simulink model "stg2_tv"  (Simulink 7.0)
settings: Solver=ode45  StartTime=0.0  StopTime=200000  RelTol=1e-3
undefined symbols (not defined in the file): pfb_coeff_gen_calc
libraries: xbsIndex_r4 x911, casper_library x87, xps_library x7
(part 1 of 12)
settings Model: Creator=dave  LastModifiedBy=dave

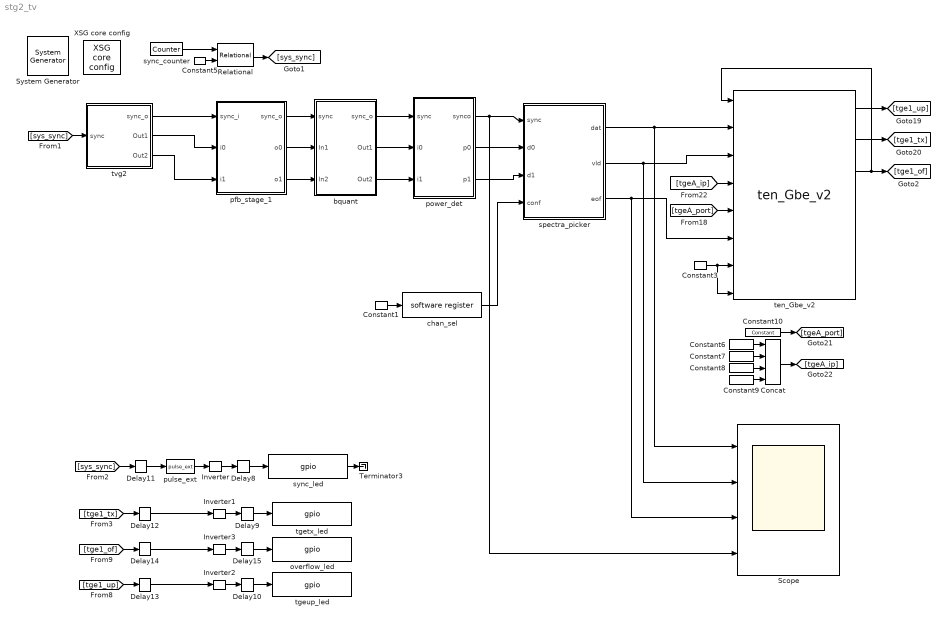
== system stg2_tv ==
  " System Generator" : xbsIndex_r4/ System Generator  Tag=genX  SystemSampleTime=-1  xilinxfamily=virtex5  part=xc5vlx110t  speed=-1  package=ff1136  synthesis_tool=XST  clock_wrapper=Clock Enables  directory=./qdr_cturn/sysgen  testbench=off  simulink_period=1  sysclk_period=8.3333  dcm_input_clock_period=100  incr_netlist=off  trim_vbits=Everywhere in SubSystem  dbl_ovrd=According to Block Masks  core_generation=According to Block Masks  run_coregen=off  deprecated_control=off  eval_field=0  block_type=sysgen
      settings: block_version=10.1.3
  Concat : xbsIndex_r4/Concat  num_inputs=4  dbl_ovrd=off  block_type=concat
      settings: block_version=10.1.3
  Constant1 : xbsIndex_r4/Constant  arith_type=Unsigned  const=4  n_bits=32  bin_pt=0  explicit_period=on  period=1  equ=P=C  opselect=C  inp2=PCIN>>17  opr=+  inp1=P  carry=CIN  dbl_ovrd=off  block_type=constant
  Constant10 : xbsIndex_r4/Constant  arith_type=Unsigned  const=10000  n_bits=16  bin_pt=0  explicit_period=off  period=1  equ=P=C  opselect=C  inp2=PCIN>>17  opr=+  inp1=P  carry=CIN  dbl_ovrd=off  block_type=constant
  Constant3 : xbsIndex_r4/Constant  arith_type=Boolean  const=0  n_bits=32  bin_pt=0  explicit_period=on  period=1  equ=P=C  opselect=C  inp2=PCIN>>17  opr=+  inp1=P  carry=CIN  dbl_ovrd=off  block_type=constant
  Constant5 : xbsIndex_r4/Constant  arith_type=Unsigned  const=0  n_bits=32  bin_pt=0  explicit_period=on  period=1  equ=P=C  opselect=C  inp2=PCIN>>17  opr=+  inp1=P  carry=CIN  dbl_ovrd=off  block_type=constant
  Constant6 : xbsIndex_r4/Constant  arith_type=Unsigned  const=192  n_bits=8  bin_pt=0  explicit_period=off  period=1  equ=P=C  opselect=C  inp2=PCIN>>17  opr=+  inp1=P  carry=CIN  dbl_ovrd=off  block_type=constant
  Constant7 : xbsIndex_r4/Constant  arith_type=Unsigned  const=168  n_bits=8  bin_pt=0  explicit_period=off  period=1  equ=P=C  opselect=C  inp2=PCIN>>17  opr=+  inp1=P  carry=CIN  dbl_ovrd=off  block_type=constant
  Constant8 : xbsIndex_r4/Constant  arith_type=Unsigned  const=5  n_bits=8  bin_pt=0  explicit_period=off  period=1  equ=P=C  opselect=C  inp2=PCIN>>17  opr=+  inp1=P  carry=CIN  dbl_ovrd=off  block_type=constant
  Constant9 : xbsIndex_r4/Constant  arith_type=Unsigned  const=2  n_bits=8  bin_pt=0  explicit_period=off  period=1  equ=P=C  opselect=C  inp2=PCIN>>17  opr=+  inp1=P  carry=CIN  dbl_ovrd=off  block_type=constant
  Delay{8..15} (8 alike) : xbsIndex_r4/Delay  en=off  latency=1  dbl_ovrd=off  reg_retiming=off  block_type=delay
  Inverter{,1..3} (4 alike) : xbsIndex_r4/Inverter  en=off  latency=0  dbl_ovrd=off  block_type=inv
  Relational : xbsIndex_r4/Relational  mode=a=b  en=off  latency=1  dbl_ovrd=off  block_type=relational
      settings: block_version=10.1.3
  Scope : Scope  NumInputPorts=4
      settings: YMin=-5~-5~-5~-5  YMax=5~5~5~5
  Terminator3 : Terminator
  XSG core config : xps_library/XSG core config  Tag=xps:xsg  SystemSampleTime=-1  hw_sys=ROACH:lx110t  ibob_linux=off  clk_src=sys_clk  iBOB_clk_src=sys_clk  BEE2_ctrl_clk_src=sys_clk  BEE2_usr_clk_src=sys_clk  ROACH_clk_src=sys_clk  CORR_clk_src=sys_clk  gpio_clk_io_group=iBOB:sma  gpio_clk_bit_index=0  clk_rate=100  sample_period=1  synthesis_tool=XST  mpc_type=powerpc440_ext
  bquant : Subsystem  mask{fact=8, bits=9}
      mask prompts: fact "fact (2^n)"; bits "quant bits"
  chan_sel : xps_library/software register  Tag=xps:sw_reg  SystemSampleTime=-1  io_dir=From Processor  arith_type=Unsigned  bitwidth=32  bin_pt=0  sample_period=1  gw_name=stg2_tv_chan_sel_user_data_out
      link override stg2_tv_chan_sel_user_data_out: arith_type=Unsigned  n_bits=32  bin_pt=0  period=1
  overflow_led : xps_library/gpio  Tag=xps:gpio  SystemSampleTime=-1  io_group=ROACH:led  io_dir=out  arith_type=Boolean  bitwidth=1  bin_pt=0  bit_index=2  sample_period=1  use_single_ended=off  use_ddr=off  reg_iob=on  reg_clk_phase=0  termination=None
      link override convert: arith_type=Boolean  n_bits=1  bin_pt=0
  pfb_stage_1 : Subsystem
  power_det : Subsystem
  pulse_ext : casper_library/Misc/pulse_ext  SystemSampleTime=-1  pulse_len=2^25
  spectra_picker : Subsystem
  sync_counter : xbsIndex_r4/Counter  cnt_type=Free Running  cnt_to=Inf  operation=Up  start_count=0  cnt_by_val=1  arith_type=Unsigned  n_bits=33  bin_pt=0  load_pin=off  rst=off  en=off  explicit_period=on  period=1  dbl_ovrd=off  use_behavioral_HDL=off  use_rpm=off  implementation=Fabric  block_type=counter
  sync_led : xps_library/gpio  Tag=xps:gpio  SystemSampleTime=-1  io_group=ROACH:led  io_dir=out  arith_type=Boolean  bitwidth=1  bin_pt=0  bit_index=0  sample_period=1  use_single_ended=off  use_ddr=off  reg_iob=on  reg_clk_phase=0  termination=None
      link override convert: arith_type=Boolean  n_bits=1  bin_pt=0
  ten_Gbe_v2 : xps_library/ten_Gbe_v2  Tag=xps:tengbe_v2  SystemSampleTime=-1  port=0  rx_dist_ram=on  show_param=on  pre_emph=3  swing=800  fab_en=on  fab_mac=hex2dec('123456780000')  fab_ip=192*(2^24) + 168*(2^16) + 5*(2^8) + 20*(2^0)  fab_udp=10000  fab_gate=1  cpu_rx_en=on  cpu_tx_en=on
  tgetx_led : xps_library/gpio  Tag=xps:gpio  SystemSampleTime=-1  io_group=ROACH:led  io_dir=out  arith_type=Boolean  bitwidth=1  bin_pt=0  bit_index=1  sample_period=1  use_single_ended=off  use_ddr=off  reg_iob=on  reg_clk_phase=0  termination=None
      link override convert: arith_type=Boolean  n_bits=1  bin_pt=0
  tgeup_led : xps_library/gpio  Tag=xps:gpio  SystemSampleTime=-1  io_group=ROACH:led  io_dir=out  arith_type=Boolean  bitwidth=1  bin_pt=0  bit_index=3  sample_period=1  use_single_ended=off  use_ddr=off  reg_iob=on  reg_clk_phase=0  termination=None
      link override convert: arith_type=Boolean  n_bits=1  bin_pt=0
  tvg2 : Subsystem
  wires:
  pulse_ext/1 -> Inverter/1
  [sys_sync] -> Delay11/1
  Delay8/1 -> sync_led/1
  Delay11/1 -> pulse_ext/1
  Inverter/1 -> Delay8/1
  sync_counter/1 -> Relational/1
  Constant5/1 -> Relational/2
  Relational/1 -> [sys_sync]
  sync_led/1 -> Terminator3/1
  [sys_sync] -> tvg2/1(sync)
  tvg2/1(sync_o) -> pfb_stage_1/1(sync_i)
  tvg2/2(Out1) -> pfb_stage_1/2(i0)
  tvg2/3(Out2) -> pfb_stage_1/3(i1)
  pfb_stage_1/1(sync_o) -> bquant/1(sync)
  pfb_stage_1/2(o0) -> bquant/2(In1)
  pfb_stage_1/3(o1) -> bquant/3(In2)
  bquant/1(sync_o) -> power_det/1(sync)
  bquant/2(Out1) -> power_det/2(i0)
  bquant/3(Out2) -> power_det/3(i1)
  Constant1/1 -> chan_sel/1
  ten_Gbe_v2/5 -> ten_Gbe_v2/1, [tge1_of]
  Constant6/1 -> Concat/1
  Constant7/1 -> Concat/2
  Constant8/1 -> Concat/3
  Constant9/1 -> Concat/4
  Concat/1 -> [tgeA_ip]
  Constant10/1 -> [tgeA_port]
  [tge1_tx] -> Delay12/1
  [tge1_up] -> Delay13/1
  Delay9/1 -> tgetx_led/1
  Delay10/1 -> tgeup_led/1
  Delay12/1 -> Inverter1/1
  Delay13/1 -> Inverter2/1
  Inverter1/1 -> Delay9/1
  Inverter2/1 -> Delay10/1
  Delay15/1 -> overflow_led/1
  Inverter3/1 -> Delay15/1
  [tge1_of] -> Delay14/1
  Delay14/1 -> Inverter3/1
  [tgeA_ip] -> ten_Gbe_v2/4
  [tgeA_port] -> ten_Gbe_v2/5
  Constant3/1 -> ten_Gbe_v2/7, ten_Gbe_v2/8
  ten_Gbe_v2/1 -> [tge1_up]
  ten_Gbe_v2/3 -> [tge1_tx]
  power_det/1(synco) -> spectra_picker/1(sync), Scope/4
  power_det/2(p0) -> spectra_picker/2(d0)
  power_det/3(p1) -> spectra_picker/3(d1)
  chan_sel/1 -> spectra_picker/4(conf)
  spectra_picker/1(dat) -> ten_Gbe_v2/2, Scope/1
  spectra_picker/2(vld) -> ten_Gbe_v2/3, Scope/2
  spectra_picker/3(eof) -> ten_Gbe_v2/6, Scope/3

== system stg2_tv/bquant ==
  sync : Inport
  In1 : Inport  Port=2
  In2 : Inport  Port=3
  Convert{,1..3} (4 alike) : xbsIndex_r4/Convert  arith_type="Signed  (2's comp)"  n_bits=bits  bin_pt=bits-1  quantization="Round  (unbiased: +/- Inf)"  overflow=Saturate  latency=0  dbl_ovrd=off  pipeline=off  block_type=convert
      settings: block_version=10.1.3
  Delay{1..5,7} (6 alike) : xbsIndex_r4/Delay  en=off  latency=1  dbl_ovrd=off  reg_retiming=off  block_type=delay
  Shift{,1..3} (4 alike) : xbsIndex_r4/Shift  shift_dir=Left  shift_bits=fact  en=off  latency=1  precision=Full  arith_type="Signed  (2's comp)"  n_bits=16  bin_pt=14  quantization=Truncate  overflow=Wrap  dbl_ovrd=off  block_type=shift
      settings: block_version=10.1.3
  c_to_ri : casper_library/Misc/c_to_ri  SystemSampleTime=-1  n_bits=25  bin_pt=24
      settings: AttributesFormatString=25_24 r/i
  c_to_ri1 : casper_library/Misc/c_to_ri  SystemSampleTime=-1  n_bits=25  bin_pt=24
      settings: AttributesFormatString=25_24 r/i
  ri_to_c : casper_library/Misc/ri_to_c  SystemSampleTime=-1
  ri_to_c1 : casper_library/Misc/ri_to_c  SystemSampleTime=-1
  sync_o : Outport
  Out1 : Outport  Port=2
  Out2 : Outport  Port=3
  wires:
  Delay3/1 -> sync_o/1
  Delay5/1 -> Delay3/1
  sync/1 -> Delay5/1
  ri_to_c1/1 -> Out2/1
  In2/1 -> c_to_ri1/1
  ri_to_c/1 -> Out1/1
  In1/1 -> c_to_ri/1
  Delay7/1 -> ri_to_c1/2
  Delay4/1 -> ri_to_c1/1
  Delay2/1 -> ri_to_c/2
  Delay1/1 -> ri_to_c/1
  Convert3/1 -> Delay7/1
  Convert2/1 -> Delay4/1
  Convert1/1 -> Delay2/1
  Convert/1 -> Delay1/1
  c_to_ri1/2 -> Shift3/1
  c_to_ri1/1 -> Shift2/1
  Shift3/1 -> Convert3/1
  Shift2/1 -> Convert2/1
  c_to_ri/2 -> Shift1/1
  c_to_ri/1 -> Shift/1
  Shift1/1 -> Convert1/1
  Shift/1 -> Convert/1

== system stg2_tv/pfb_stage_1 ==
  sync_i : Inport
  i0 : Inport  Port=2
  i1 : Inport  Port=3
  " window" : Subsystem  mask{wintype=0, size=10, coeff_width=18, o_width=25, i_width=9}
      mask prompts: wintype "Windowing Function:"; size "size (2^n)"; coeff_width "coeff width"; o_width "out width"; i_width "in width"
  Constant4 : xbsIndex_r4/Constant  arith_type=Unsigned  const=1023  n_bits=10  bin_pt=0  explicit_period=on  period=1  equ=P=C  opselect=C  inp2=PCIN>>17  opr=+  inp1=P  carry=CIN  dbl_ovrd=off  block_type=constant
  Delay{,1..3} (4 alike) : xbsIndex_r4/Delay  en=off  latency=1  dbl_ovrd=off  reg_retiming=off  block_type=delay
  Shift{1..4} (4 alike) : xbsIndex_r4/Shift  shift_dir=Right  shift_bits=1  en=off  latency=1  precision=Full  arith_type="Signed  (2's comp)"  n_bits=16  bin_pt=14  quantization=Truncate  overflow=Wrap  dbl_ovrd=off  block_type=shift
      settings: block_version=10.1.3
  c_to_ri : casper_library/Misc/c_to_ri  SystemSampleTime=-1  n_bits=25  bin_pt=24
      settings: AttributesFormatString=25_24 r/i
  c_to_ri1 : casper_library/Misc/c_to_ri  SystemSampleTime=-1  n_bits=25  bin_pt=24
      settings: AttributesFormatString=25_24 r/i
  fft : Subsystem  AncestorBlock=casper_library/FFTs/fft  mask(fft){FFTSize=10, input_bit_width=25, coeff_bit_width=18, n_inputs=0, quantization=Truncate, overflow=Wrap, add_latency=1, mult_latency=3, bram_latency=3, arch=Virtex5, opt_target=Multipliers, coeffs_bit_limit=8, delays_bit_limit=9, specify_mult=off, mult_spec=[0 1 1 2 1 1 1 1 1 1]}
      mask prompts: FFTSize "Size of FFT: (2^?)"; input_bit_width "Input/Output Bit Width"; coeff_bit_width "Coefficient Bit Width"; n_inputs "Number of Simultaneous Inputs: (2^?)"; quantization "Quantization Behavior"; overflow "Overflow Behavior"; add_latency "Add Latency"; mult_latency "Mult Latency"; bram_latency "BRAM Latency"; arch "Architecture"; opt_target "Optimisation Target"; coeffs_bit_limit "Number bits above which to store stage's coefficients in BRAM (2^? bits)"; delays_bit_limit "Number bits above which to store stage's delays in BRAM (2^? bits)"; specify_mult "Specify multiplier use (behavioral HDL if not specified)"; mult_spec "Multiplier specification (0=core, 1=embedded, 2=behavioural) (left=1st stage)"
      mask init:
      | fft_init(gcb,...
      |     'FFTSize', FFTSize, ...
      |     'input_bit_width', input_bit_width, ...
      |     'coeff_bit_width', coeff_bit_width, ...
      |     'n_inputs', n_inputs, ...
      |     'quantization', quantization, ...
      |     'overflow', overflow, ...
      |     'add_latency', add_latency, ...
      |     'mult_latency', mult_latency, ...
      |     'bram_latency', bram_latency, ...
      |     'arch', arch, ...
      |     'opt_target', opt_target, ...
      |     'coeffs_bit_limit', coeffs_bit_limit, ...
      |     'delays_bit_limit', delays_bit_limit, ...
      |     'specify_mult', specify_mult, ...
      |     'mult_spec', mult_spec);
      settings: AttributesFormatString=FFTSize=10, n_inputs=0
      mask Help: eval('xlWeb([getenv(''MLIB_ROOT''), ''\doc\htmlblocks\sp_fft\sp_fft.html''])')
      mask StyleString: edit,edit,edit,edit,popup(Truncate|Round  (unbiased: +/- Inf)|Round  (unbiased: Even Values)),popup(Wrap|Saturate|Error),edit,edit,edit,popup(Virtex2Pro|Virtex5),popup(Logic|Multipliers),edit,edit,checkbox,edit
      mask CallbackString:
      | % fft_size = eval(get_param(gcb, 'FFTSize'));
      | % old_vec = eval(get_param(gcb, 'mult_spec'));
      | 
      | % vec = 2.*ones(1,fft_size);
      | % old_size = length(old_vec);
      | 
      | % if(old_size <= fft_size), size = old_size;
      | % else, size = fft_size;
      | % end
      | 
      | % for n = 1:size, vec(n) = old_vec(n); end
      | % set_param(gcb, 'mult_spec', mat2str(vec));|||||||||||||specify_mult = get_param(gcb,'specify_mult');
      | visibs = get_param(gcb, 'MaskVisibilities');
      | if( strcmp(specify_mult,'off')), visibs{15} = 'off';
      | else visibs{15} = 'on';
      | end
      | set_param(gcb, 'MaskVisibilities', visibs);
      | 
      | |% vec = eval( get_param(gcb, 'mult_spec'));
      | % vec_size = length(vec);
      | % fft_size = eval( get_param(gcb, 'FFTSize'));
      | % new_vec = 2.*ones(1, fft_size);
      | 
      | % if(vec_size <= fft_size), size = vec_size;
      | % else size = fft_size;
      | % end
      | 
      | % for n=1:size,
      | %    new_vec(n) = vec(n);
      | % end
      | % set_param(gcb, 'mult_spec', mat2str(new_vec));
  ri_to_c : casper_library/Misc/ri_to_c  SystemSampleTime=-1
  ri_to_c1 : casper_library/Misc/ri_to_c  SystemSampleTime=-1
  sync_o : Outport
  o0 : Outport  Port=2
  o1 : Outport  Port=3
  wires:
  " window"/3(pol1_o) -> c_to_ri1/1
  " window"/2(pol0_o) -> c_to_ri/1
  " window"/1(sync_o) -> Delay/1
  ri_to_c1/1 -> Delay3/1
  Shift2/1 -> ri_to_c1/2
  Shift4/1 -> ri_to_c1/1
  c_to_ri1/2 -> Shift2/1
  c_to_ri1/1 -> Shift4/1
  ri_to_c/1 -> Delay2/1
  Shift1/1 -> ri_to_c/2
  Shift3/1 -> ri_to_c/1
  c_to_ri/2 -> Shift1/1
  c_to_ri/1 -> Shift3/1
  Delay/1 -> Delay1/1
  sync_i/1 -> " window"/1(sync)
  fft/3(out1) -> o1/1
  fft/2(out0) -> o0/1
  fft/1(sync_out) -> sync_o/1
  Constant4/1 -> fft/2(shift)
  i1/1 -> " window"/3(pol1_i)
  i0/1 -> " window"/2(pol0_i)
  Delay1/1 -> fft/1(sync)
  Delay2/1 -> fft/3(pol0)
  Delay3/1 -> fft/4(pol1)

== system stg2_tv/power_det ==
  sync : Inport
  i0 : Inport  Port=2
  i1 : Inport  Port=3
  Delay2 : xbsIndex_r4/Delay  en=off  latency=3  dbl_ovrd=off  reg_retiming=off  block_type=delay
  power0 : casper_library/Misc/power  SystemSampleTime=-1  BitWidth=9  add_latency=1  mult_latency=2
  power1 : casper_library/Misc/power  SystemSampleTime=-1  BitWidth=9  add_latency=1  mult_latency=2
  synco : Outport
  p0 : Outport  Port=2
  p1 : Outport  Port=3
  wires:
  Delay2/1 -> synco/1
  sync/1 -> Delay2/1
  power1/1 -> p1/1
  i1/1 -> power1/1
  power0/1 -> p0/1
  i0/1 -> power0/1

== system stg2_tv/spectra_picker ==
  sync : Inport
  d0 : Inport  Port=2
  d1 : Inport  Port=3
  conf : Inport  Port=4
  Constant2 : xbsIndex_r4/Constant  arith_type=Unsigned  const=2^10-1  n_bits=10  bin_pt=0  explicit_period=on  period=1  equ=P=C  opselect=C  inp2=PCIN>>17  opr=+  inp1=P  carry=CIN  dbl_ovrd=off  block_type=constant
  Delay{,1..4} (5 alike) : xbsIndex_r4/Delay  en=off  latency=1  dbl_ovrd=off  reg_retiming=off  block_type=delay
  Logical : xbsIndex_r4/Logical  logical_function=AND  inputs=2  en=off  latency=0  precision=Full  arith_type=Unsigned  n_bits=16  bin_pt=0  align_bp=on  dbl_ovrd=off  block_type=logical
  Mux : xbsIndex_r4/Mux  inputs=2  en=off  latency=0  precision=Full  arith_type=Unsigned  n_bits=16  bin_pt=14  quantization=Truncate  overflow=Wrap  dbl_ovrd=off  block_type=mux
  Relational1 : xbsIndex_r4/Relational  mode=a=b  en=off  latency=1  dbl_ovrd=off  block_type=relational
      settings: block_version=10.1.3
  Relational2 : xbsIndex_r4/Relational  mode=a=b  en=off  latency=1  dbl_ovrd=off  block_type=relational
      settings: block_version=10.1.3
  Slice : xbsIndex_r4/Slice  nbits=9  boolean_output=off  mode=Lower Bit Location + Width  bit1=0  base1=LSB of Input  bit0=1  base0=LSB of Input  dbl_ovrd=off  block_type=slice
      settings: infoedit="Extracts a given range of bits from each input sample and presents it at the output.  The output type is ordinarily unsigned with binary point at zero, but can be Boolean when the slice is one bit wide.<P><P>Hardware notes: In hardware this block costs nothing."  block_version=10.1.3
  Slice1 : xbsIndex_r4/Slice  nbits=1  boolean_output=off  mode=Lower Bit Location + Width  bit1=0  base1=LSB of Input  bit0=0  base0=LSB of Input  dbl_ovrd=off  block_type=slice
      settings: infoedit="Extracts a given range of bits from each input sample and presents it at the output.  The output type is ordinarily unsigned with binary point at zero, but can be Boolean when the slice is one bit wide.<P><P>Hardware notes: In hardware this block costs nothing."  block_version=10.1.3
  Slice2 : xbsIndex_r4/Slice  nbits=9  boolean_output=off  mode=Lower Bit Location + Width  bit1=0  base1=LSB of Input  bit0=10  base0=LSB of Input  dbl_ovrd=off  block_type=slice
      settings: infoedit="Extracts a given range of bits from each input sample and presents it at the output.  The output type is ordinarily unsigned with binary point at zero, but can be Boolean when the slice is one bit wide.<P><P>Hardware notes: In hardware this block costs nothing."  block_version=10.1.3
  Slice3 : xbsIndex_r4/Slice  nbits=10  boolean_output=off  mode=Lower Bit Location + Width  bit1=0  base1=LSB of Input  bit0=0  base0=LSB of Input  dbl_ovrd=off  block_type=slice
      settings: infoedit="Extracts a given range of bits from each input sample and presents it at the output.  The output type is ordinarily unsigned with binary point at zero, but can be Boolean when the slice is one bit wide.<P><P>Hardware notes: In hardware this block costs nothing."  block_version=10.1.3
  frame_counter : xbsIndex_r4/Counter  cnt_type=Free Running  cnt_to=Inf  operation=Up  start_count=0  cnt_by_val=1  arith_type=Unsigned  n_bits=19  bin_pt=0  load_pin=off  rst=on  en=off  explicit_period=on  period=1  dbl_ovrd=off  use_behavioral_HDL=off  use_rpm=off  implementation=Fabric  block_type=counter
  dat : Outport
  vld : Outport  Port=2
  eof : Outport  Port=3
  wires:
  Delay/1 -> Slice/1, Slice1/1
  Slice1/1 -> Mux/1
  frame_counter/1 -> Slice2/1, Slice3/1
  Slice2/1 -> Relational1/1
  Slice/1 -> Relational1/2
  Mux/1 -> Delay1/1
  Slice3/1 -> Relational2/1
  Constant2/1 -> Relational2/2
  Relational2/1 -> Logical/1
  Relational1/1 -> Logical/2, Delay3/1
  Logical/1 -> Delay2/1
  Delay1/1 -> Delay4/1
  sync/1 -> frame_counter/1
  d0/1 -> Mux/2
  d1/1 -> Mux/3
  Delay2/1 -> eof/1
  Delay3/1 -> vld/1
  conf/1 -> Delay/1
  Delay4/1 -> dat/1

== system stg2_tv/tvg2 ==
  sync : Inport  OutDataType=sfix(16)  OutScaling=2^0
  Constant : xbsIndex_r4/Constant  arith_type=Signed (2's comp)  const=0  n_bits=9  bin_pt=8  explicit_period=on  period=1  equ=P=C  opselect=C  inp2=PCIN>>17  opr=+  inp1=P  carry=CIN  dbl_ovrd=off  block_type=constant
  Delay : xbsIndex_r4/Delay  en=off  latency=1  dbl_ovrd=off  reg_retiming=off  block_type=delay
  Delay1 : xbsIndex_r4/Delay  en=off  latency=1  dbl_ovrd=off  reg_retiming=off  block_type=delay
  Delay2 : xbsIndex_r4/Delay  en=off  latency=3  dbl_ovrd=off  reg_retiming=off  block_type=delay
  Delay3 : xbsIndex_r4/Delay  en=off  latency=1  dbl_ovrd=off  reg_retiming=off  block_type=delay
  Delay4 : xbsIndex_r4/Delay  en=off  latency=2  dbl_ovrd=off  reg_retiming=off  block_type=delay
  Mult : xbsIndex_r4/Mult  precision=User Defined  arith_type=Unsigned  n_bits=12  bin_pt=0  quantization=Truncate  overflow=Wrap  en=off  latency=3  dbl_ovrd=off  use_behavioral_HDL=off  use_embedded=on  opt=Speed  optimum_pipeline=off  pipeline=on  use_rpm=on  placement_style=Triangular  block_type=mult
      settings: infoedit=Hardware notes: To use the internal pipeline stage of the dedicated multiplier you must select 'Pipeline for maximum performance'.  block_version=10.1.3
  Shift : xbsIndex_r4/Shift  shift_dir=Right  shift_bits=6  en=off  latency=1  precision=User Defined  arith_type="Signed  (2's comp)"  n_bits=9  bin_pt=8  quantization="Round  (unbiased: +/- Inf)"  overflow=Wrap  dbl_ovrd=off  block_type=shift
      settings: block_version=10.1.3
  chan_s : xbsIndex_r4/Slice  nbits=9  boolean_output=off  mode=Lower Bit Location + Width  bit1=0  base1=LSB of Input  bit0=10  base0=LSB of Input  dbl_ovrd=off  block_type=slice
      settings: infoedit="Extracts a given range of bits from each input sample and presents it at the output.  The output type is ordinarily unsigned with binary point at zero, but can be Boolean when the slice is one bit wide.<P><P>Hardware notes: In hardware this block costs nothing."  block_version=10.1.3
  chan_s1 : xbsIndex_r4/Slice  nbits=10  boolean_output=off  mode=Lower Bit Location + Width  bit1=0  base1=LSB of Input  bit0=0  base0=LSB of Input  dbl_ovrd=off  block_type=slice
      settings: infoedit="Extracts a given range of bits from each input sample and presents it at the output.  The output type is ordinarily unsigned with binary point at zero, but can be Boolean when the slice is one bit wide.<P><P>Hardware notes: In hardware this block costs nothing."  block_version=10.1.3
  progress : xbsIndex_r4/Counter  cnt_type=Free Running  cnt_to=Inf  operation=Up  start_count=0  cnt_by_val=1  arith_type=Unsigned  n_bits=19  bin_pt=0  load_pin=off  rst=on  en=off  explicit_period=on  period=1  dbl_ovrd=off  use_behavioral_HDL=off  use_rpm=off  implementation=Fabric  block_type=counter
  ri_to_c : casper_library/Misc/ri_to_c  SystemSampleTime=-1
  ri_to_c1 : casper_library/Misc/ri_to_c  SystemSampleTime=-1
  tvg_lookup : xbsIndex_r4/ROM  depth=4096  initVector=cos(pi*(0:4065)/128)  distributed_mem=Block RAM  rst=off  init_reg=0  en=off  latency=2  arith_type="Signed  (2's comp)"  n_bits=9  bin_pt=8  dbl_ovrd=off  optimize=Area  use_rpm=on  block_type=sprom
      settings: block_version=10.1.3
  sync_o : Outport
  Out1 : Outport  Port=2
  Out2 : Outport  Port=3
  wires:
  progress/1 -> chan_s/1, chan_s1/1
  chan_s/1 -> [chan]
  chan_s1/1 -> [samp]
  ri_to_c/1 -> Out1/1
  ri_to_c1/1 -> Out2/1
  Constant/1 -> ri_to_c/2, ri_to_c1/1
  tvg_lookup/1 -> Shift/1
  Delay/1 -> ri_to_c/1, ri_to_c1/2
  sync/1 -> progress/1, Delay2/1
  Delay3/1 -> Delay1/1
  Delay1/1 -> sync_o/1
  [chan] -> Mult/1
  [samp] -> Mult/2
  Mult/1 -> tvg_lookup/1
  Delay2/1 -> Delay4/1
  Shift/1 -> Delay/1
  Delay4/1 -> Delay3/1

== system stg2_tv/pfb_stage_1/ window ==
  sync : Inport
  pol0_i : Inport  Port=2
  pol1_i : Inport  Port=3
  Delay : xbsIndex_r4/Delay  en=off  latency=2  dbl_ovrd=off  reg_retiming=off  block_type=delay
  Delay1 : xbsIndex_r4/Delay  en=off  latency=3  dbl_ovrd=off  reg_retiming=off  block_type=delay
  Mult{,1..3} (4 alike) : xbsIndex_r4/Mult  precision=Full  arith_type="Signed  (2's comp)"  n_bits=16  bin_pt=14  quantization=Truncate  overflow=Wrap  en=off  latency=3  dbl_ovrd=off  use_behavioral_HDL=off  use_embedded=on  opt=Speed  optimum_pipeline=off  pipeline=on  use_rpm=on  placement_style=Triangular  block_type=mult
      settings: infoedit=Hardware notes: To use the internal pipeline stage of the dedicated multiplier you must select 'Pipeline for maximum performance'.  block_version=10.1.3
  c_to_ri : casper_library/Misc/c_to_ri  SystemSampleTime=-1  n_bits=i_width  bin_pt=i_width-1
      settings: AttributesFormatString=9_8 r/i
  c_to_ri1 : casper_library/Misc/c_to_ri  SystemSampleTime=-1  n_bits=i_width  bin_pt=i_width-1
      settings: AttributesFormatString=9_8 r/i
  lookup_cntr : xbsIndex_r4/Counter  cnt_type=Free Running  cnt_to=Inf  operation=Up  start_count=0  cnt_by_val=1  arith_type=Unsigned  n_bits=size  bin_pt=0  load_pin=off  rst=on  en=off  explicit_period=on  period=1  dbl_ovrd=off  use_behavioral_HDL=off  use_rpm=off  implementation=Fabric  block_type=counter
  ri_to_c : casper_library/Misc/ri_to_c  SystemSampleTime=-1
  ri_to_c1 : casper_library/Misc/ri_to_c  SystemSampleTime=-1
  window_lookup : xbsIndex_r4/ROM  depth=2^size  initVector=pfb_coeff_gen_calc(size, 1,'hamming',0, 0,1,1)  distributed_mem=Block RAM  rst=off  init_reg=0  en=off  latency=2  arith_type="Signed  (2's comp)"  n_bits=18  bin_pt=17  dbl_ovrd=off  optimize=Area  use_rpm=on  block_type=sprom
      settings: block_version=10.1.3
  sync_o : Outport
  pol0_o : Outport  Port=2
  pol1_o : Outport  Port=3
  wires:
  Delay/1 -> Delay1/1
  lookup_cntr/1 -> window_lookup/1
  sync/1 -> lookup_cntr/1, Delay/1
  pol0_i/1 -> c_to_ri/1
  window_lookup/1 -> Mult/1, Mult1/1, Mult2/1, Mult3/1
  c_to_ri/1 -> Mult/2
  c_to_ri/2 -> Mult1/2
  Delay1/1 -> sync_o/1
  Mult/1 -> ri_to_c/1
  Mult1/1 -> ri_to_c/2
  Mult2/1 -> ri_to_c1/1
  Mult3/1 -> ri_to_c1/2
  pol1_i/1 -> c_to_ri1/1
  c_to_ri1/1 -> Mult2/2
  c_to_ri1/2 -> Mult3/2
  ri_to_c/1 -> pol0_o/1
  ri_to_c1/1 -> pol1_o/1

== system stg2_tv/pfb_stage_1/fft ==
  sync : Inport  OutDataType=sfix(16)  OutScaling=2^0
  shift : Inport  Port=2  OutDataType=sfix(16)  OutScaling=2^0
  pol0 : Inport  Port=3
  pol1 : Inport  Port=4
  fft_biplex0 : Subsystem  AncestorBlock=casper_library/FFTs/fft_biplex  mask(fft_biplex){FFTSize=10, input_bit_width=25, coeff_bit_width=18, quantization=Truncate, overflow=Wrap, add_latency=1, mult_latency=3, bram_latency=3, arch=Virtex5, opt_target=Multipliers, coeffs_bit_limit=8, delays_bit_limit=9, specify_mult=off, mult_spec=[2 2 2 2 2 2 2 2 2 2]}
      mask prompts: FFTSize "Size of FFT: (2^? pnts)"; input_bit_width "Input/Output Bit Width"; coeff_bit_width "Coefficient Bit Width"; quantization "Quantization Behavior"; overflow "Overflow Behavior"; add_latency "Add Latency"; mult_latency "Mult Latency"; bram_latency "BRAM Latency"; arch "Architecture"; opt_target "Optimisation Target"; coeffs_bit_limit "Number bits above which to store stage's coefficients in BRAM (2^? bits)"; delays_bit_limit "Number bits above which to implent stage's delays in BRAM (2^? bits)"; specify_mult "Specify multiplier use (behavioral HDL if not specified)"; mult_spec "Multiplier specification (0=core, 1=embedded, 2=behavioural) (left=1st stage)"
      mask init:
      | fft_biplex_init(gcb,...
      |     'FFTSize', FFTSize,...
      |     'input_bit_width', input_bit_width,...
      |     'coeff_bit_width', coeff_bit_width,...
      |     'quantization', quantization,...
      |     'overflow', overflow,...
      |     'add_latency', add_latency,...
      |     'mult_latency', mult_latency,...
      |     'bram_latency', bram_latency,...
      |     'arch', arch, ...
      |     'opt_target', opt_target, ...
      |     'coeffs_bit_limit', coeffs_bit_limit, ...
      |     'delays_bit_limit', delays_bit_limit, ...
      |     'specify_mult', specify_mult,...
      |     'mult_spec', mult_spec);
      settings: AttributesFormatString=|
      | FFTSize=10,
      |  arch=Virtex5,
      |  opt_target=Multipliers
      mask StyleString: edit,edit,edit,popup(Truncate|Round  (unbiased: +/- Inf)|Round  (unbiased: Even Values)),popup(Wrap|Saturate|Error),edit,edit,edit,popup(Virtex2Pro|Virtex5),popup(Logic|Multipliers),edit,edit,checkbox,edit
      mask CallbackString:
      | % fft_size = eval(get_param(gcb, 'FFTSize'));
      | % old_vec = eval(get_param(gcb, 'mult_spec'));
      | 
      | % vec = 2.*ones(1,fft_size);
      | % old_size = length(old_vec);
      | 
      | % if(old_size <= fft_size),
      | %    size = old_size;
      | % else,
      | %     size = fft_size;
      | % end
      | 
      | % for n = 1:size, vec(n) = old_vec(n); end
      | % set_param(gcb, 'mult_spec', mat2str(vec));||||||||||||specify_mult = get_param(gcb,'specify_mult');
      | visibs = get_param(gcb, 'MaskVisibilities');
      | 
      | if( strcmp(specify_mult,'off')), visibs{14} = 'off';
      | else, visibs{14} = 'on';
      | end
      | set_param(gcb, 'MaskVisibilities', visibs);
      | |% vec = eval( get_param(gcb, 'mult_spec'));
      | % vec_size = length(vec);
      | % fft_size = eval( get_param(gcb, 'FFTSize'));
      | % new_vec = 2.*ones(1, fft_size);
      | 
      | % if(vec_size <= fft_size), size = vec_size;
      | % else size = fft_size;
      | % end
      | 
      | % for n=1:size
      | %     new_vec(n) = vec(n);
      | % end
      | % set_param(gcb, 'mult_spec', mat2str(new_vec));
  sync_out : Outport
  out0 : Outport  Port=2
  out1 : Outport  Port=3
  of : Outport  Port=4
  wires:
  pol0/1 -> fft_biplex0/1(pol1)
  pol1/1 -> fft_biplex0/2(pol2)
  shift/1 -> fft_biplex0/4(shift)
  sync/1 -> fft_biplex0/3(sync)
  fft_biplex0/1(pol1_out) -> out0/1
  fft_biplex0/2(pol2_out) -> out1/1
  fft_biplex0/4(sync_out) -> sync_out/1
  fft_biplex0/3(of) -> of/1

== system stg2_tv/pfb_stage_1/fft/fft_biplex0 ==
  pol1 : Inport  OutDataType=sfix(16)  OutScaling=2^0
  pol2 : Inport  Port=2  OutDataType=sfix(16)  OutScaling=2^0
  sync : Inport  Port=3  OutDataType=sfix(16)  OutScaling=2^0
  shift : Inport  Port=4  OutDataType=sfix(16)  OutScaling=2^0
  biplex_core : Subsystem  AncestorBlock=casper_library/FFTs/biplex_core  mask(biplex_core){FFTSize=10, input_bit_width=25, coeff_bit_width=18, quantization=Truncate, overflow=Wrap, add_latency=1, mult_latency=3, bram_latency=3, arch=Virtex5, opt_target=Multipliers, coeffs_bit_limit=8, delays_bit_limit=9, specify_mult=off, mult_spec=[2 2 2 2 2 2 2 2 2 2]}
      mask prompts: FFTSize "Size of FFT: (2^? pnts)"; input_bit_width "Input/Output Bit Width"; coeff_bit_width "Coefficient Bit Width"; quantization "Quantization Behavior"; overflow "Overflow Behavior"; add_latency "Add Latency"; mult_latency "Mult Latency"; bram_latency "BRAM Latency"; arch "Architecture"; opt_target "Optimisation Target"; coeffs_bit_limit "Number bits above which to store stage's coefficients in BRAM (2^? bits)"; delays_bit_limit "Number bits above which to implent stage's delays in BRAM (2^? bits)"; specify_mult "Specify multiplier use (behavioural HDL if not specified)"; mult_spec "Multiplier specification (0=core, 1=embedded, 2=behavioural) (left=1st stage)"
      mask init:
      | biplex_core_init(gcb,...
      |     'FFTSize', FFTSize,...
      |     'input_bit_width', input_bit_width,...
      |     'coeff_bit_width', coeff_bit_width,...
      |     'quantization', quantization,...
      |     'overflow', overflow,...
      |     'add_latency', add_latency,...
      |     'mult_latency', mult_latency,...
      |     'bram_latency', bram_latency,...
      |     'arch', arch, ...
      |     'opt_target', opt_target, ...
      |     'coeffs_bit_limit', coeffs_bit_limit, ...
      |     'delays_bit_limit', delays_bit_limit, ...
      |     'specify_mult', specify_mult,...
      |     'mult_spec', mult_spec);
      settings: AttributesFormatString=|
      | FFTSize=10,
      |  opt_target=Multipliers,
      |  arch=Virtex5
      mask StyleString: edit,edit,edit,popup(Truncate|Round  (unbiased: +/- Inf)|Round  (unbiased: Even Values)),popup(Wrap|Saturate|Error),edit,edit,edit,popup(Virtex2Pro|Virtex5),popup(Logic|Multipliers),edit,edit,checkbox,edit
      mask CallbackString:
      | fft_size = eval(get_param(gcb, 'FFTSize'));
      | old_vec = eval(get_param(gcb, 'mult_spec'));
      | 
      | vec = 2.*ones(1,fft_size);
      | old_size = length(old_vec);
      | 
      | if(old_size <= fft_size),
      |     size = old_size;
      | else,
      |     size = fft_size;
      | end
      | 
      | for n = 1:size, vec(n) = old_vec(n); end
      | set_param(gcb, 'mult_spec', mat2str(vec));||||||||||||specify_mult = get_param(gcb,'specify_mult');
      | visibs = get_param(gcb,'MaskVisibilities');
      | if( strcmp(specify_mult,'off')), visibs{14} = 'off';
      | else, visibs{14} = 'on';
      | end
      | set_param(gcb, 'MaskVisibilities', visibs);
      | enables = get_param(gcb,'MaskVisibilities');
      | enables{14} = 'on';
      | set_param(gcb, 'MaskEnables', enables);
      | |vec = eval( get_param(gcb, 'mult_spec'));
      | vec_size = length(vec);
      | fft_size = eval( get_param(gcb, 'FFTSize'));
      | new_vec = 2.*ones(1, fft_size);
      | 
      | if(vec_size <= fft_size), size = vec_size;
      | else size = fft_size;
      | end
      | 
      | for n=1:size
      |     new_vec(n) = vec(n);
      | end
      | set_param(gcb, 'mult_spec', mat2str(new_vec));
  biplex_cplx_unscrambler : Subsystem  mask{FFTSize=10, bram_latency=3}
      mask prompts: FFTSize "Size of FFT: (2^? pnts)"; bram_latency "BRAM Latency"
      mask init:
      | blk = gcb;
      | if same_state(blk, 'FFTSize', FFTSize, 'bram_latency', bram_latency), return, end
      | map = bit_reverse(0:2^(FFTSize-1)-1, FFTSize-1);
      | set_param([blk,'/reorder'],'map',mat2str([map,map+2^(FFTSize-1)]));
      | set_param([blk,'/reorder'],'bram_latency', num2str(bram_latency));
      | set_param([blk,'/reorder1'],'map',mat2str([map+2^(FFTSize-1),map]));
      | set_param([blk,'/reorder1'],'bram_latency', num2str(bram_latency));
      | save_state(blk, 'FFTSize', FFTSize, 'bram_latency', bram_latency);
  pol1_out : Outport  OutDataType=sfix(16)  OutScaling=2^0
  pol2_out : Outport  Port=2  OutDataType=sfix(16)  OutScaling=2^0
  of : Outport  Port=3  OutDataType=sfix(16)  OutScaling=2^0
  sync_out : Outport  Port=4  OutDataType=sfix(16)  OutScaling=2^0
  wires:
  biplex_cplx_unscrambler/3(sync_out) -> sync_out/1
  biplex_cplx_unscrambler/2(pol2) -> pol2_out/1
  biplex_core/4(sync_out) -> biplex_cplx_unscrambler/3(sync)
  biplex_core/2(out2) -> biplex_cplx_unscrambler/2(odd)
  biplex_core/1(out1) -> biplex_cplx_unscrambler/1(even)
  pol1/1 -> biplex_core/1(pol1)
  pol2/1 -> biplex_core/2(pol2)
  sync/1 -> biplex_core/3(sync)
  shift/1 -> biplex_core/4(shift)
  biplex_cplx_unscrambler/1(pol1) -> pol1_out/1
  biplex_core/3(of) -> of/1
